simulink model "TST_DYN_2018b"  (Simulink 9.2)
settings: Solver=ode45  StartTime=0.0  StopTime="sim_par.t_end  "  MaxStep="sim_par.t_step "  RelTol=sim_par.rel_solver_tol
libraries: DYN x1, POSTPROC x1
settings Model: Creator=alger  LastModifiedBy=Mike  SimulationMode=rapid-accelerator
settings DataIOCC: LimitDataPoints=off  SaveFormat=Dataset  SignalLoggingSaveFormat=Dataset
settings OptimizationCC: LifeSpan=auto
settings DebuggingCC: UnderspecifiedInitializationDetection=Simplified  MergeDetectMultiDrivingBlocksExec=error  FcnCallInpInsideContextMsg=error  StateNameClashWarn=none  SFUnexpectedBacktrackingDiag=error  SFNoUnconditionalDefaultTransitionDiag=error  SFExecutionAtInitializationDiag=warning
settings HardwareCC: ProdBitPerPointer=64  ProdBitPerSizeT=64  ProdBitPerPtrDiffT=64  ProdLargestAtomicFloat=Float  ProdIntDivRoundTo=Zero  ProdEndianess=LittleEndian  ProdWordSize=64  ProdHWDeviceType=Intel->x86-64 (Windows64)
settings ModelReferenceCC: PropagateSignalLabelsOutOfModel=on
settings GRTTargetCC: TargetLangStandard=C99 (ISO)  GeneratePreprocessorConditionals=Use local settings  CombineOutputUpdateFcns=on  GRTInterface=off
settings ConfigComp: CovMetricSettings=dwe  CovHtmlReporting=off  CovSaveCumulativeToWorkspaceVar=off  CovSaveSingleToWorkspaceVar=off  CovExternalEMLEnable=on

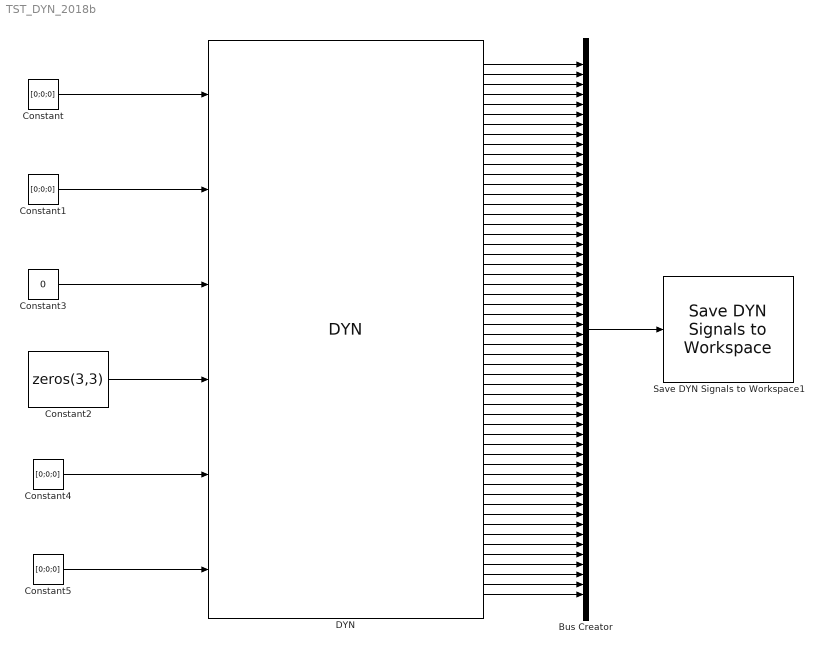
== system TST_DYN_2018b ==
  Bus Creator : BusCreator  Inputs=54
  Constant{,1,4..5} (4 alike) : Constant  Value=[0;0;0]
  Constant2 : Constant  Value=zeros(3,3)
  Constant3 : Constant  Value=0
  DYN : DYN/DYN  SystemSampleTime=-1  Latency=0  AutoFrameSizeCalculation=off
  Save DYN Signals to Workspace1 : POSTPROC/Save DYN Signals to Workspace  SystemSampleTime=-1  Latency=0  AutoFrameSizeCalculation=off
  wires:
  DYN/45 -> Bus Creator/45
  DYN/2 -> Bus Creator/2
  DYN/12 -> Bus Creator/12
  DYN/47 -> Bus Creator/47
  DYN/34 -> Bus Creator/34
  DYN/6 -> Bus Creator/6
  DYN/27 -> Bus Creator/27
  DYN/17 -> Bus Creator/17
  DYN/20 -> Bus Creator/20
  DYN/40 -> Bus Creator/40
  DYN/44 -> Bus Creator/44
  DYN/7 -> Bus Creator/7
  DYN/23 -> Bus Creator/23
  DYN/8 -> Bus Creator/8
  DYN/4 -> Bus Creator/4
  DYN/25 -> Bus Creator/25
  DYN/9 -> Bus Creator/9
  DYN/13 -> Bus Creator/13
  DYN/19 -> Bus Creator/19
  DYN/24 -> Bus Creator/24
  DYN/28 -> Bus Creator/28
  DYN/32 -> Bus Creator/32
  DYN/36 -> Bus Creator/36
  DYN/10 -> Bus Creator/10
  DYN/18 -> Bus Creator/18
  DYN/26 -> Bus Creator/26
  DYN/38 -> Bus Creator/38
  DYN/1 -> Bus Creator/1
  DYN/39 -> Bus Creator/39
  DYN/43 -> Bus Creator/43
  DYN/15 -> Bus Creator/15
  DYN/22 -> Bus Creator/22
  DYN/46 -> Bus Creator/46
  DYN/37 -> Bus Creator/37
  DYN/11 -> Bus Creator/11
  DYN/5 -> Bus Creator/5
  DYN/29 -> Bus Creator/29
  DYN/16 -> Bus Creator/16
  DYN/30 -> Bus Creator/30
  DYN/14 -> Bus Creator/14
  DYN/21 -> Bus Creator/21
  DYN/31 -> Bus Creator/31
  DYN/3 -> Bus Creator/3
  DYN/33 -> Bus Creator/33
  DYN/35 -> Bus Creator/35
  DYN/41 -> Bus Creator/41
  DYN/42 -> Bus Creator/42
  Constant/1 -> DYN/1
  Constant1/1 -> DYN/2
  Constant2/1 -> DYN/4
  Constant3/1 -> DYN/3
  Bus Creator/1 -> Save DYN Signals to Workspace1/1
  DYN/48 -> Bus Creator/48
  DYN/49 -> Bus Creator/49
  DYN/50 -> Bus Creator/50
  DYN/51 -> Bus Creator/51
  DYN/52 -> Bus Creator/52
  DYN/53 -> Bus Creator/53
  Constant4/1 -> DYN/5
  Constant5/1 -> DYN/6
  DYN/54 -> Bus Creator/54
